simulink model "lab001"  (R2020b)
settings: Solver=VariableStepAuto  StartTime=0.0  StopTime=10.0  RelTol=1e-3
settings Model: Creator=karth  LastModifiedBy=karth

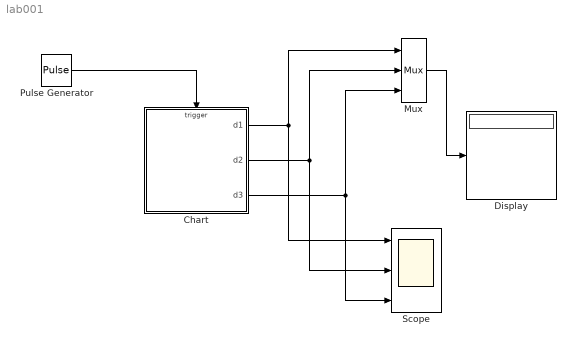
== system lab001 ==
  Chart : Stateflow chart  TreatAsAtomicUnit=on
  Display : Display
  Mux : Mux  Inputs=3
  Pulse Generator : DiscretePulseGenerator  PulseType=Time based  Period=10  PulseWidth=5
  Scope : Scope  NumInputPorts=3
  wires:
  Mux/1 -> Display/1
  Pulse Generator/1 -> Chart/Trigger
  Chart/3(d3) -> Mux/3, Scope/3
  Chart/2(d2) -> Mux/2, Scope/2
  Chart/1(d1) -> Mux/1, Scope/1

== stateflow chart lab001/Chart ==
  state digit1 [parallel]
    settings: executionOrder=1
    state zero
      en:d1=0;
    state one
      en:d1=1;
    state two
      en:d1=2;
    state three
      en:d1=3;
    state four
      en:d1=4;
    (default) -> digit1.zero
    digit1.zero -> digit1.one : inpclick
    digit1.one -> digit1.two : inpclick
    digit1.two -> digit1.three : inpclick
    digit1.three -> digit1.four : inpclick
    digit1.four -> digit1.zero : inpclick/{digit2.inc2}
  state digit2 [parallel]
    settings: executionOrder=2
    state zero
      en:d2=0;
    state one
      en:d2=1;
    state two
      en:d2=2;
    state three
      en:d2=3;
    state four
      en:d2=4;
    (default) -> digit2.zero
    digit2.zero -> digit2.one : inc2
    digit2.one -> digit2.two : inc2
    digit2.two -> digit2.three : inc2
    digit2.three -> digit2.four : inc2
    digit2.four -> digit2.zero : inc2/{digit3.inc3}
  state digit3 [parallel]
    settings: executionOrder=3
    state zero
      en:d3=0;
    state one
      en:d3=1;
    state two
      en:d3=2;
    state three
      en:d3=3;
    state four
      en:d3=4;
    (default) -> digit3.zero
    digit3.zero -> digit3.one : inc3
    digit3.one -> digit3.two : inc3
    digit3.two -> digit3.three : inc3
    digit3.three -> digit3.four : inc3
    digit3.four -> digit3.zero : inc3
  data: d1 output; d2 output; d3 output
  events: inc2 local FUNCTION_CALL_EVENT; inc3 local FUNCTION_CALL_EVENT; inpclick input RISING_EDGE_EVENT
